simulink model "simulink9"  (R2025b)
settings: Solver=ode45  StartTime=0.0  StopTime=150  MaxStep=0.05  RelTol=1e-3
libraries: simulink x2
settings Model: Creator=mizula  LastModifiedBy=mizula

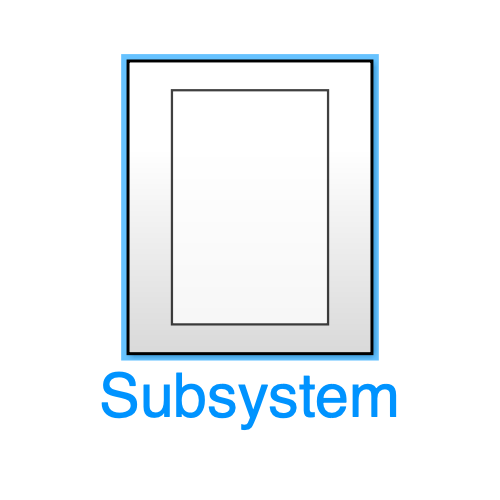
[thumbnail: Simulink's stored preview of the top-level diagram]
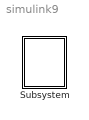
== system simulink9 ==
  Subsystem : Subsystem

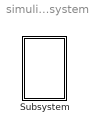
== system simulink9/Subsystem ==
  Subsystem : Subsystem  mask{h1=4, h2=2, S1=1, S2=2, Swy1=0.2, Swy2=0.2, fi1=1, fi2=1, g=9.81, Qwe=2}

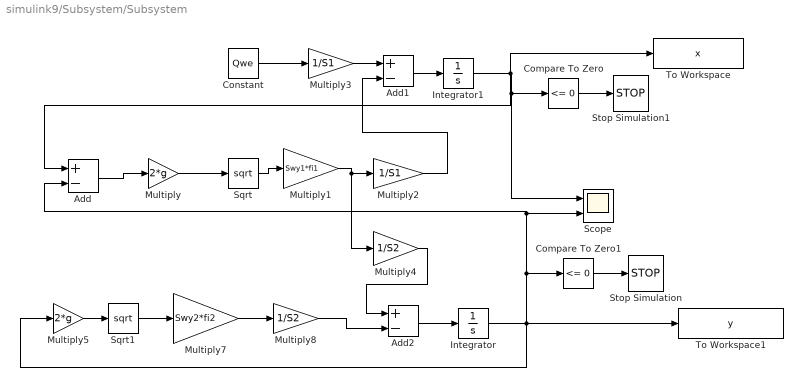
== system simulink9/Subsystem/Subsystem ==
  Add : Sum  Inputs=+-
  Add1 : Sum  Inputs=+-
  Add2 : Sum  Inputs=+-
  Compare To Zero : simulink/Logic and Bit Operations/Compare To Zero  relop=<=  OutDataTypeStr=boolean
  Compare To Zero1 : simulink/Logic and Bit Operations/Compare To Zero  relop=<=  OutDataTypeStr=boolean
  Constant : Constant  Value=Qwe
  Integrator : Integrator  InitialCondition=h2
  Integrator1 : Integrator  InitialCondition=h1
  Multiply : Gain  Gain=2*g
  Multiply1 : Gain  Gain=Swy1*fi1
  Multiply2 : Gain  Gain=1/S1
  Multiply3 : Gain  Gain=1/S1
  Multiply4 : Gain  Gain=1/S2
  Multiply5 : Gain  Gain=2*g
  Multiply7 : Gain  Gain=Swy2*fi2
  Multiply8 : Gain  Gain=1/S2
  Scope : Scope  NumInputPorts=2
      settings: ActiveDisplayYMinimum=-1  ActiveDisplayYMaximum=1
  Sqrt : Sqrt
  Sqrt1 : Sqrt
  Stop Simulation : Stop
  Stop Simulation1 : Stop
  To Workspace : ToWorkspace  VariableName=x  SaveFormat=Timeseries  SampleTime=-1
  To Workspace1 : ToWorkspace  VariableName=y  SaveFormat=Timeseries  SampleTime=-1
  wires:
  Multiply/1 -> Sqrt/1
  Multiply3/1 -> Add1/1
  Add1/1 -> Integrator1/1
  Multiply2/1 -> Add1/2
  Multiply1/1 -> Multiply4/1, Multiply2/1
  Constant/1 -> Multiply3/1
  Compare To Zero1/1 -> Stop Simulation/1
  Multiply7/1 -> Multiply8/1
  Add2/1 -> Integrator/1
  Multiply4/1 -> Add2/1
  Multiply8/1 -> Add2/2
  Integrator/1 -> Compare To Zero1/1, Add/2, Scope/2, Multiply5/1, To Workspace1/1
  Sqrt/1 -> Multiply1/1
  Add/1 -> Multiply/1
  Integrator1/1 -> To Workspace/1, Add/1, Scope/1, Compare To Zero/1
  Compare To Zero/1 -> Stop Simulation1/1
  Multiply5/1 -> Sqrt1/1
  Sqrt1/1 -> Multiply7/1
